simulink model "PowerFetDCmotor"  (R2014a)
settings: Solver=ode15s  StartTime=0.0  StopTime=1  RelTol=1e-3
libraries: elec_lib x13, fl_lib x13, nesl_utility x5
settings Model: Creator=laca  LastModifiedBy=laca
settings DebuggingCC: UnderspecifiedInitializationDetection=Classic

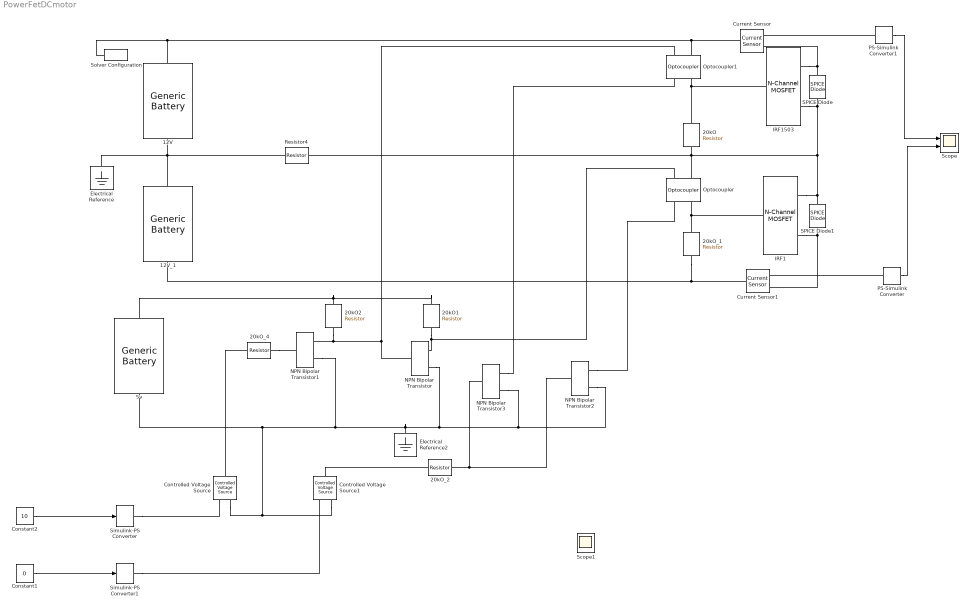
== system PowerFetDCmotor ==
  12V : elec_lib/Sources/Generic Battery  Vnom=12 V  R1=0.1 Ohm  prm_AH=1  AH=50 hr*A  AH0=50 hr*A  V1=11.5 V  AH1=25 hr*A  prm_R2=1  R2=2e+3 Ohm
  12V_1 : elec_lib/Sources/Generic Battery  Vnom=12 V  R1=0.1 Ohm  prm_AH=1  AH=50 hr*A  AH0=50 hr*A  V1=11.5 V  AH1=25 hr*A  prm_R2=1  R2=2e+3 Ohm
  20kO : fl_lib/Electrical/Electrical Elements/Resistor  R=20 kOhm  i_specify=off  i_priority=High  i=0 A  v_specify=on  v_priority=High  v=0 V
  20kO1 : fl_lib/Electrical/Electrical Elements/Resistor  R=10 Ohm  i_specify=off  i_priority=High  i=0 A  v_specify=on  v_priority=High  v=0 V
  20kO2 : fl_lib/Electrical/Electrical Elements/Resistor  R=10 Ohm  i_specify=off  i_priority=High  i=0 A  v_specify=on  v_priority=High  v=0 V
  20kO_1 : fl_lib/Electrical/Electrical Elements/Resistor  R=20 kOhm  i_specify=off  i_priority=High  i=0 A  v_specify=on  v_priority=High  v=0 V
  20kO_2 : fl_lib/Electrical/Electrical Elements/Resistor  R=2000 Ohm  i_specify=off  i_priority=High  i=0 A  v_specify=off  v_priority=High  v=0 V
  20kO_4 : fl_lib/Electrical/Electrical Elements/Resistor  R=20 Ohm  i_specify=off  i_priority=High  i=0 A  v_specify=off  v_priority=High  v=0 V
  5v : elec_lib/Sources/Generic Battery  Vnom=5 V  R1=0.1 Ohm  prm_AH=1  AH=50 hr*A  AH0=50 hr*A  V1=11.5 V  AH1=25 hr*A  prm_R2=1  R2=2e+3 Ohm
  Constant1 : Constant  Value=0
  Constant2 : Constant  Value=10
  Controlled Voltage Source : fl_lib/Electrical/Electrical Sources/Controlled Voltage Source
  Controlled Voltage Source1 : fl_lib/Electrical/Electrical Sources/Controlled Voltage Source
  Current Sensor : fl_lib/Electrical/Electrical Sensors/Current Sensor
  Current Sensor1 : fl_lib/Electrical/Electrical Sensors/Current Sensor
  Electrical Reference : fl_lib/Electrical/Electrical Elements/Electrical Reference
  Electrical Reference2 : fl_lib/Electrical/Electrical Elements/Electrical Reference
  IRF1 : elec_lib/Semiconductor Devices/N-Channel MOSFET  parameterization=1  prmDatasheet=1  prmEquCoeff=1  Beta=5 A/V^2  Rds=0.0033 Ohm  Id=75 A  Vgs=10 V  Vth=3 V  lam=0 1/V  Tmeas=25 C  RS=1e-4 Ohm  RD=0.001 Ohm  C_param=1  C_GS=270 pF  C_GD=80 pF  C_iss=5730 pF  C_rss=290 pF  C_oss=2250 pF  charge_linearity_param=1  C_OX=200 pF  V_C_OX=-0.5 V  dVth_dT=-6 mV/K  Rds_T2=0.037 Ohm  Tmeas2=125 C  BEXDatasheet=-1.5  BEXEquCoeff=-1.5  TdeviceDatasheet=25 C  TdeviceEquCoeff=25 C  Rth=[ 0 10 ] K/W  thermal_mass_parameterization=1  thermal_mass=[ 0 1 ] J/K  thermal_time_constant=[ 0 10 ] s  thermal_mass_initial_temperatures=[ 25 25 ] C
  IRF1503 : elec_lib/Semiconductor Devices/N-Channel MOSFET  parameterization=1  prmDatasheet=1  prmEquCoeff=1  Beta=5 A/V^2  Rds=0.0033 Ohm  Id=75 A  Vgs=10 V  Vth=3 V  lam=0 1/V  Tmeas=25 C  RS=1e-4 Ohm  RD=0.001 Ohm  C_param=1  C_GS=270 pF  C_GD=80 pF  C_iss=5730 pF  C_rss=290 pF  C_oss=2250 pF  charge_linearity_param=1  C_OX=200 pF  V_C_OX=-0.5 V  dVth_dT=-6 mV/K  Rds_T2=0.037 Ohm  Tmeas2=125 C  BEXDatasheet=-1.5  BEXEquCoeff=-1.5  TdeviceDatasheet=25 C  TdeviceEquCoeff=25 C  Rth=[ 0 10 ] K/W  thermal_mass_parameterization=1  thermal_mass=[ 0 1 ] J/K  thermal_time_constant=[ 0 10 ] s  thermal_mass_initial_temperatures=[ 25 25 ] C
  NPN Bipolar Transistor{,1..3} (4 alike) : elec_lib/Semiconductor Devices/NPN Bipolar Transistor  parameterization=1  prmDatasheet=1  prmEquCoeff=1  BF=100  IS=1e-14 A  ec=1  VAF=200 V  hfe=100  hoe=5e-5 1/Ohm  Ic_h=1 mA  Vce_h=5 V  V1=0.55 V  I1=0.5 mA  BR=1  Tmeas=25 C  RC=0.01 Ohm  RE=1e-4 Ohm  RB=1 Ohm  C_BC=5 pF  C_BE=5 pF  TF=0 us  TR=0 us  hfe_T2=125  XTB=0  V1_T2=0.45 V  I1_T2=0.5 mA  Tmeas2=125 C  EG=1.11 eV  XTI=3  TdeviceDatasheet=25 C  TdeviceEquCoeff=25 C  Rth=[ 0 10 ] K/W  thermal_mass_parameterization=1  thermal_mass=[ 0 1 ] J/K  thermal_time_constant=[ 0 10 ] s  thermal_mass_initial_temperatures=[ 25 25 ] C
  Optocoupler : elec_lib/Semiconductor Devices/Optocoupler  CTR=0.2  prmExp=2  I12=[ 0.001 0.015 ] A  V12=[ 0.9 1.05 ] V  RS=0.1 Ohm  IS=1e-10 A  Tmeas=25 C  ec=2  C_param=1  CJ0=5 pF  VJ=1 V  Mgrad=0.5  Vvec=[ 0.1 10 100 ] V  Cvec=[ 3.5 1 0.4 ] pF  FC=0.5  T_param=1  IS_T2=1.8e-8 A  I1_T2=0.029 A  V1_T2=1.05 V  Tmeas2=125 C  EG_param=1  EG=1.11 eV  XTI_param=1  XTI=3  Tdevice=25 C  Rth=[ 0 10 ] K/W  thermal_mass_parameterization=1  thermal_mass=[ 0 1 ] J/K  thermal_time_constant=[ 0 10 ] s  thermal_mass_initial_temperatures=[ 25 25 ] C
  Optocoupler1 : elec_lib/Semiconductor Devices/Optocoupler  CTR=0.2  prmExp=2  I12=[ 0.001 0.015 ] A  V12=[ 0.9 1.05 ] V  RS=0.1 Ohm  IS=1e-10 A  Tmeas=25 C  ec=2  C_param=1  CJ0=5 pF  VJ=1 V  Mgrad=0.5  Vvec=[ 0.1 10 100 ] V  Cvec=[ 3.5 1 0.4 ] pF  FC=0.5  T_param=1  IS_T2=1.8e-8 A  I1_T2=0.029 A  V1_T2=1.05 V  Tmeas2=125 C  EG_param=1  EG=1.11 eV  XTI_param=1  XTI=3  Tdevice=25 C  Rth=[ 0 10 ] K/W  thermal_mass_parameterization=1  thermal_mass=[ 0 1 ] J/K  thermal_time_constant=[ 0 10 ] s  thermal_mass_initial_temperatures=[ 25 25 ] C
  PS-Simulink Converter : nesl_utility/PS-Simulink Converter  PhysicalDomain=network_engine_domain  SubClassName=ps_output  LeftPortType=input  RightPortType=output  PseudoPeriodic=off  Frequencies=[]  Unit=1  AffineConversion=off
  PS-Simulink Converter1 : nesl_utility/PS-Simulink Converter  PhysicalDomain=network_engine_domain  SubClassName=ps_output  LeftPortType=input  RightPortType=output  PseudoPeriodic=off  Frequencies=[]  Unit=1  AffineConversion=off
  Resistor4 : fl_lib/Electrical/Electrical Elements/Resistor  R=1 Ohm  i_specify=off  i_priority=High  i=0 A  v_specify=on  v_priority=High  v=0 V
  SPICE Diode : elec_lib/Additional Components/SPICE-Compatible Components/Semiconductor Devices/SPICE Diode  AREA=1 m^2  SCALE=1  IS=1e-14 A/m^2  RS=0.01 m^2*Ohm  ND=1  C_param=1  CJO=0 F/m^2  VJ=1 V  MG=0.5  FC=0.5  TT=0 s  RevBrk=1  BV=Inf V  IBV=0.001 A/m^2  T_param=1  XTI=3  EG=1.11 eV  TOFFSET=0 K  TFIXED=300.15 K  TMEAS=300.15 K  IC_given=1  V0=0 V
  SPICE Diode1 : elec_lib/Additional Components/SPICE-Compatible Components/Semiconductor Devices/SPICE Diode  AREA=1 m^2  SCALE=1  IS=1e-14 A/m^2  RS=0.01 m^2*Ohm  ND=1  C_param=1  CJO=0 F/m^2  VJ=1 V  MG=0.5  FC=0.5  TT=0 s  RevBrk=1  BV=Inf V  IBV=0.001 A/m^2  T_param=1  XTI=3  EG=1.11 eV  TOFFSET=0 K  TFIXED=300.15 K  TMEAS=300.15 K  IC_given=1  V0=0 V
  Scope : Scope  NumInputPorts=2
      settings: YMin=10.8757~-2.28767e-11  YMax=10.8757~-2.28767e-11
  Scope1 : Scope  NumInputPorts=2
      settings: YMin=1.14001e-11~-1.26e-11  YMax=1.26001e-11~-1.14e-11
  Simulink-PS Converter : nesl_utility/Simulink-PS Converter  PhysicalDomain=network_engine_domain  SubClassName=ps_input  LeftPortType=input  RightPortType=output  PseudoPeriodic=off  Frequencies=[]  NoiseDistribution=none  NoiseParameters=[]  Unit=1  AffineConversion=off  InputFiltering=off  SimscapeFilterOrder=1  InputFilterTimeConstant=0.001  UdotUserProvided=1
  Simulink-PS Converter1 : nesl_utility/Simulink-PS Converter  PhysicalDomain=network_engine_domain  SubClassName=ps_input  LeftPortType=input  RightPortType=output  PseudoPeriodic=off  Frequencies=[]  NoiseDistribution=none  NoiseParameters=[]  Unit=1  AffineConversion=off  InputFiltering=off  SimscapeFilterOrder=1  InputFilterTimeConstant=0.001  UdotUserProvided=1
  Solver Configuration : nesl_utility/Solver Configuration  PhysicalDomain=network_engine_domain  SubClassName=solver  LeftPortType=input  RightPortType=generic  Accelerate=off  Tones=[]  Harmonics=[]  SimulateNoise=off  Profile=off  UseLocalSampling=off  EnableSwitchedLinearOptims=on  FrequencyDomain=off  UseCCode=off  RelTol=0.001  AbsTol=1e-06  MinStep=1e-09  ToWorkspace=off  DoDC=on  ResidualTolerance=1e-9  UseLocalSolver=on  LocalSolverChoice=NE_TRAPEZOIDAL_ADVANCER  LocalSolverSampleTime=.01  DoFixedCost=off  MaxNonlinIter=3  MaxModeIter=2  LinearAlgebra=Sparse  DelaysMemoryBudget=1024  AutomaticFiltering=on  FilteringTimeConstant=0.001
  wires:
  Constant2/1 -> Simulink-PS Converter/1
  PS-Simulink Converter1/1 -> Scope/1
  PS-Simulink Converter/1 -> Scope/2
  Constant1/1 -> Simulink-PS Converter1/1
  connections:
  Solver Configuration/RConn1 -- Optocoupler1/LConn2 -- Current Sensor/LConn1 -- 12V/LConn1
  12V/RConn1 -- Electrical Reference/LConn1 -- 12V_1/LConn1 -- Resistor4/RConn1
  SPICE Diode1/RConn1 -- IRF1/RConn1 -- IRF1503/RConn2 -- SPICE Diode/LConn1 -- 20kO/RConn1 -- Optocoupler/LConn2 -- Resistor4/LConn1
  Simulink-PS Converter/RConn1 -- Controlled Voltage Source/RConn1
  Simulink-PS Converter1/RConn1 -- Controlled Voltage Source1/RConn1
  PS-Simulink Converter/LConn1 -- Current Sensor1/RConn1
  PS-Simulink Converter1/LConn1 -- Current Sensor/RConn1
  20kO1/RConn1 -- Optocoupler/LConn1 -- NPN Bipolar Transistor/RConn1
  IRF1503/RConn1 -- SPICE Diode/RConn1 -- Current Sensor/RConn2
  Current Sensor1/LConn1 -- 20kO_1/RConn1 -- 12V_1/RConn1
  20kO2/RConn1 -- Optocoupler1/LConn1 -- NPN Bipolar Transistor/LConn1 -- NPN Bipolar Transistor1/RConn1
  20kO_1/LConn1 -- Optocoupler/RConn2 -- IRF1/LConn1
  NPN Bipolar Transistor2/RConn2 -- NPN Bipolar Transistor3/RConn2 -- NPN Bipolar Transistor/RConn2 -- Electrical Reference2/LConn1 -- NPN Bipolar Transistor1/RConn2 -- Controlled Voltage Source/RConn2 -- Controlled Voltage Source1/RConn2 -- 5v/RConn1
  20kO_4/LConn1 -- NPN Bipolar Transistor1/LConn1
  20kO1/LConn1 -- 20kO2/LConn1 -- 5v/LConn1
  NPN Bipolar Transistor2/RConn1 -- Optocoupler/RConn1
  NPN Bipolar Transistor3/RConn1 -- Optocoupler1/RConn1
  NPN Bipolar Transistor3/LConn1 -- NPN Bipolar Transistor2/LConn1 -- 20kO_2/RConn1
  Controlled Voltage Source/LConn1 -- 20kO_4/RConn1
  Controlled Voltage Source1/LConn1 -- 20kO_2/LConn1
  Optocoupler1/RConn2 -- 20kO/LConn1 -- IRF1503/LConn1
  SPICE Diode1/LConn1 -- IRF1/RConn2 -- Current Sensor1/RConn2
